simulink model "ARINC429_BNR"  (R2020b)
settings: Solver=VariableStepAuto  StartTime=0.0  StopTime=10.0  RelTol=1e-3
libraries: Bibavion x1
(part 1 of 3)
settings Model: Creator=Nicolas  LastModifiedBy=rolla

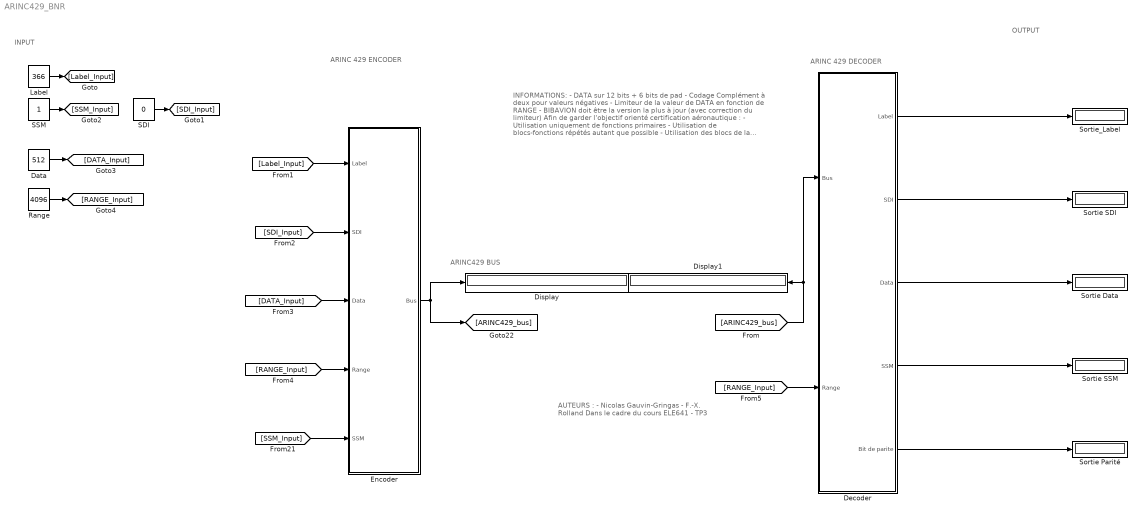
== system ARINC429_BNR ==
  note: AUTEURS :
      | - Nicolas Gauvin-Gringas
      | - F.-X. Rolland
      |
      | Dans le cadre du cours ELE641 - TP3
  note: INFORMATIONS:
      | - DATA sur 12 bits + 6 bits de pad
      | - Codage Complément à deux pour valeurs négatives
      | - Limiteur de la valeur de DATA en fonction de RANGE
      | - BIBAVION doit être la version la plus à jour (avec correction du limiteur)
      |
      | Afin de garder l'objectif orienté certification aéronautique :
      | - Utilisation uniquement de fonctions primaires
      | - Utilisation de blocs-fonctions répétés autant que possible
      | - Utilisation des blocs de la fonction BIBAVION partout la où possible
  note: ARINC 429 DECODER
  note: ARINC 429 ENCODER
  note: ARINC429 BUS
  note: OUTPUT
  note: INPUT
  Data : Constant  Value=512  OutDataTypeStr=int32  SampleTime=-1
  Decoder : Subsystem
  Display : Display
      settings: Format=binary (Stored Integer)
  Display1 : Display
      settings: Format=binary (Stored Integer)
  Encoder : Subsystem
  Label : Constant  Value=366  OutDataTypeStr=uint32  SampleTime=-1
  Range : Constant  Value=4096  OutDataTypeStr=uint32  SampleTime=-1
  SDI : Constant  Value=0  OutDataTypeStr=uint32  SampleTime=-1
  SSM : Constant  OutDataTypeStr=uint32  SampleTime=-1
  Sortie Data : Display
  Sortie Parité : Display
  Sortie SDI : Display
  Sortie SSM : Display
  Sortie_Label : Display
  wires:
  [ARINC429_bus] -> Decoder/1(Bus), Display1/1
  Label/1 -> [Label_Input]
  SDI/1 -> [SDI_Input]
  SSM/1 -> [SSM_Input]
  Decoder/1(Label) -> Sortie_Label/1
  [Label_Input] -> Encoder/1(Label)
  Encoder/1(Bus) -> Display/1, [ARINC429_bus]
  [SDI_Input] -> Encoder/2(SDI)
  [SSM_Input] -> Encoder/5(SSM)
  Decoder/2(SDI) -> Sortie SDI/1
  Decoder/3(Data) -> Sortie Data/1
  Decoder/4(SSM) -> Sortie SSM/1
  Decoder/5(Bit de parite) -> Sortie Parité/1
  Range/1 -> [RANGE_Input]
  [RANGE_Input] -> Encoder/4(Range)
  Data/1 -> [DATA_Input]
  [DATA_Input] -> Encoder/3(Data)
  [RANGE_Input] -> Decoder/2(Range)

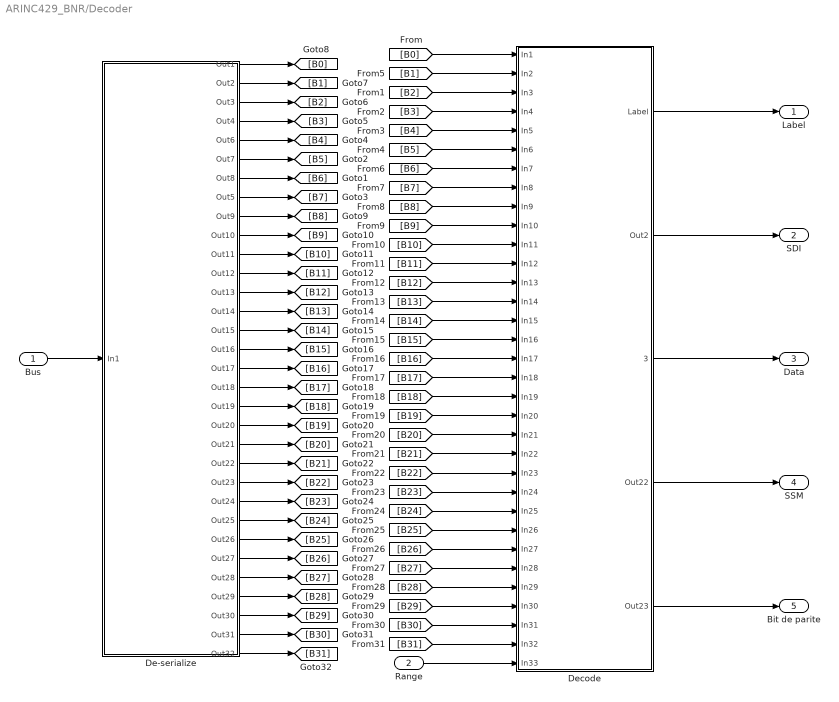
== system ARINC429_BNR/Decoder ==
  Bus : Inport
  Range : Inport  Port=2
  De-serialize : Subsystem
  Decode : Subsystem
  Label : Outport
  SDI : Outport  Port=2
  Data : Outport  Port=3
  SSM : Outport  Port=4
  Bit de parite : Outport  Port=5
  wires:
  De-serialize/6(Out7) -> [B5]
  De-serialize/1(Out1) -> [B0]
  De-serialize/7(Out8) -> [B6]
  De-serialize/5(Out6) -> [B4]
  De-serialize/3(Out3) -> [B2]
  De-serialize/2(Out2) -> [B1]
  De-serialize/4(Out4) -> [B3]
  De-serialize/8(Out5) -> [B7]
  Bus/1 -> De-serialize/1(In1)
  [B1] -> Decode/2(In2)
  [B0] -> Decode/1(In1)
  [B2] -> Decode/3(In3)
  [B3] -> Decode/4(In4)
  [B4] -> Decode/5(In5)
  [B5] -> Decode/6(In6)
  [B6] -> Decode/7(In7)
  [B7] -> Decode/8(In8)
  De-serialize/9(Out9) -> [B8]
  De-serialize/10(Out10) -> [B9]
  De-serialize/11(Out11) -> [B10]
  De-serialize/12(Out12) -> [B11]
  De-serialize/13(Out13) -> [B12]
  De-serialize/14(Out14) -> [B13]
  De-serialize/15(Out15) -> [B14]
  De-serialize/16(Out16) -> [B15]
  De-serialize/17(Out17) -> [B16]
  De-serialize/18(Out18) -> [B17]
  De-serialize/19(Out19) -> [B18]
  De-serialize/20(Out20) -> [B19]
  De-serialize/21(Out21) -> [B20]
  De-serialize/22(Out22) -> [B21]
  De-serialize/23(Out23) -> [B22]
  De-serialize/24(Out24) -> [B23]
  De-serialize/25(Out25) -> [B24]
  De-serialize/26(Out26) -> [B25]
  De-serialize/27(Out27) -> [B26]
  De-serialize/28(Out28) -> [B27]
  De-serialize/29(Out29) -> [B28]
  De-serialize/30(Out30) -> [B29]
  De-serialize/31(Out31) -> [B30]
  De-serialize/32(Out32) -> [B31]
  [B8] -> Decode/9(In9)
  [B9] -> Decode/10(In10)
  [B10] -> Decode/11(In11)
  [B11] -> Decode/12(In12)
  [B12] -> Decode/13(In13)
  [B13] -> Decode/14(In14)
  [B14] -> Decode/15(In15)
  [B15] -> Decode/16(In16)
  [B16] -> Decode/17(In17)
  [B17] -> Decode/18(In18)
  [B18] -> Decode/19(In19)
  [B19] -> Decode/20(In20)
  [B20] -> Decode/21(In21)
  [B21] -> Decode/22(In22)
  [B22] -> Decode/23(In23)
  [B23] -> Decode/24(In24)
  [B24] -> Decode/25(In25)
  [B25] -> Decode/26(In26)
  [B26] -> Decode/27(In27)
  [B27] -> Decode/28(In28)
  [B28] -> Decode/29(In29)
  [B29] -> Decode/30(In30)
  [B30] -> Decode/31(In31)
  [B31] -> Decode/32(In32)
  Decode/4(Out22) -> SSM/1
  Decode/5(Out23) -> Bit de parite/1
  Decode/2(Out2) -> SDI/1
  Decode/3(3) -> Data/1
  Range/1 -> Decode/33(In33)
  Decode/1(Label) -> Label/1

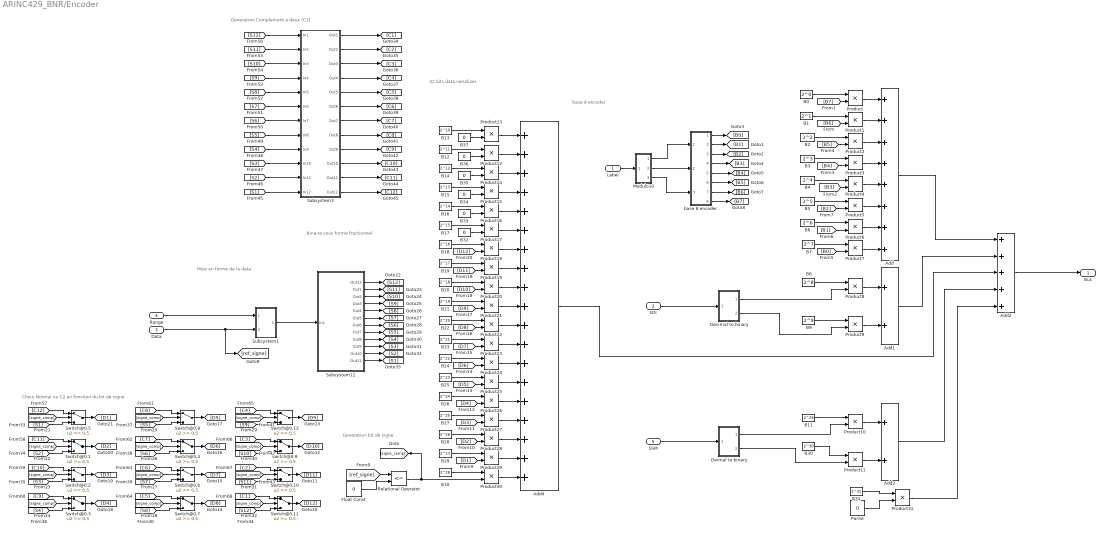
== system ARINC429_BNR/Encoder ==
  note: Generation Complement à deux (C2)
  note: Choix Normal ou C2 en fonction du bit de signe
  note: Generation bit de signe
  note: Binaire sous forme fractionnel
  note: Mise en forme de la data
  note: base 8 encoder
  note: 32 bits data serializer
  Label : Inport
  SDI : Inport  Port=2
  Data : Inport  Port=3
  Range : Inport  Port=4
  SSM : Inport  Port=5
  Add : Sum  Inputs=++++++++  AccumDataTypeStr=uint32  OutDataTypeStr=uint32
  Add1 : Sum  AccumDataTypeStr=uint32  OutDataTypeStr=uint32
  Add2 : Sum  Inputs=+++++  AccumDataTypeStr=uint32  OutDataTypeStr=uint32
  Add3 : Sum  AccumDataTypeStr=uint32  OutDataTypeStr=uint32
  Add4 : Sum  Inputs=+++++++++++++++++++  AccumDataTypeStr=uint32  OutDataTypeStr=uint32
  B0 : Constant  Value=2^0  OutDataTypeStr=single
  B1 : Constant  Value=2^1  OutDataTypeStr=single
  B10 : Constant  Value=2^28  OutDataTypeStr=single
  B11 : Constant  Value=2^29  OutDataTypeStr=single
  B12 : Constant  Value=2^11  OutDataTypeStr=single
  B13 : Constant  Value=2^10  OutDataTypeStr=single
  B14 : Constant  Value=2^12  OutDataTypeStr=single
  B15 : Constant  Value=2^13  OutDataTypeStr=single
  B16 : Constant  Value=2^14  OutDataTypeStr=single
  B17 : Constant  Value=2^15  OutDataTypeStr=single
  B18 : Constant  Value=2^16  OutDataTypeStr=single
  B19 : Constant  Value=2^17  OutDataTypeStr=single
  B2 : Constant  Value=2^2  OutDataTypeStr=single
  B20 : Constant  Value=2^18  OutDataTypeStr=single
  B21 : Constant  Value=2^19  OutDataTypeStr=single
  B22 : Constant  Value=2^20  OutDataTypeStr=single
  B23 : Constant  Value=2^21  OutDataTypeStr=single
  B24 : Constant  Value=2^22  OutDataTypeStr=single
  B25 : Constant  Value=2^23  OutDataTypeStr=single
  B26 : Constant  Value=2^24  OutDataTypeStr=single
  B27 : Constant  Value=2^25  OutDataTypeStr=single
  B28 : Constant  Value=2^26  OutDataTypeStr=single
  B29 : Constant  Value=2^27  OutDataTypeStr=single
  B3 : Constant  Value=2^3  OutDataTypeStr=single
  B30 : Constant  Value=2^30  OutDataTypeStr=single
  B31 : Constant  Value=2^31  OutDataTypeStr=single
  B{32..37} (6 alike) : Constant  Value=0  OutDataTypeStr=single
  B4 : Constant  Value=2^4  OutDataTypeStr=single
  B5 : Constant  Value=2^5  OutDataTypeStr=single
  B6 : Constant  Value=2^6  OutDataTypeStr=single
  B7 : Constant  Value=2^7  OutDataTypeStr=single
  B8 : Constant  Value=2^8  OutDataTypeStr=single
  B9 : Constant  Value=2^9  OutDataTypeStr=single
  Decimal to binary : Subsystem
  Deimal to binary : Subsystem
  Float Const : Constant  Value=0  OutDataTypeStr=uint32
  "Modulo10 " : Subsystem
  Parité : Constant  Value=0  OutDataTypeStr=boolean
  Product{,1..29,31} (31 alike) : Product
  Product30 : Product  OutDataTypeStr=single
  Relational Operator : RelationalOperator  Operator=<=  OutDataTypeStr=boolean  RndMeth=Nearest
  Subsystem1 : Subsystem
  Subsystem12 : Subsystem
  Subsystem3 : Subsystem
  Switch@0.{1..12} (12 alike) : Switch  Threshold=0.5
  base 8 encoder : Subsystem
  Bus : Outport
  wires:
  base 8 encoder/4(Out4) -> [B3]
  B5/1 -> Product5/1
  [B0] -> Product7/2
  B2/1 -> Product2/1
  [B5] -> Product2/2
  [B3] -> Product4/2
  "Modulo10 "/2(Out2) -> base 8 encoder/2(In2)
  "Modulo10 "/3(Out3) -> base 8 encoder/3(In3)
  B0/1 -> Product/1
  Product3/1 -> Add/4
  [B7] -> Product/2
  Product4/1 -> Add/5
  base 8 encoder/5(Out5) -> [B4]
  base 8 encoder/8(Out8) -> [B7]
  [B6] -> Product1/2
  B1/1 -> Product1/1
  [B4] -> Product3/2
  B4/1 -> Product4/1
  base 8 encoder/3(Out3) -> [B2]
  Product/1 -> Add/1
  Product5/1 -> Add/6
  Product6/1 -> Add/7
  base 8 encoder/1(Out1) -> [B0]
  [B1] -> Product6/2
  base 8 encoder/7(Out7) -> [B6]
  Product2/1 -> Add/3
  B3/1 -> Product3/1
  Label/1 -> "Modulo10 "/1(In1)
  Product7/1 -> Add/8
  Product1/1 -> Add/2
  B6/1 -> Product6/1
  B7/1 -> Product7/1
  "Modulo10 "/1(Out1) -> base 8 encoder/1(In1)
  base 8 encoder/6(Out6) -> [B5]
  [B2] -> Product5/2
  base 8 encoder/2(Out2) -> [B1]
  Product9/1 -> Add1/2
  Product8/1 -> Add1/1
  B9/1 -> Product9/1
  B8/1 -> Product8/1
  Product10/1 -> Add3/1
  Product11/1 -> Add3/2
  B13/1 -> Product13/1
  B12/1 -> Product12/1
  B14/1 -> Product14/1
  B15/1 -> Product15/1
  B16/1 -> Product16/1
  B17/1 -> Product17/1
  B18/1 -> Product18/1
  B19/1 -> Product19/1
  B20/1 -> Product20/1
  B21/1 -> Product21/1
  B22/1 -> Product22/1
  B23/1 -> Product23/1
  B24/1 -> Product24/1
  B25/1 -> Product25/1
  B26/1 -> Product26/1
  B27/1 -> Product27/1
  B28/1 -> Product28/1
  B29/1 -> Product29/1
  SDI/1 -> Decimal to binary/1(In1)
  Decimal to binary/1(Out1) -> Product8/2
  Decimal to binary/2(Out2) -> Product9/2
  SSM/1 -> Deimal to binary/1(In1)
  Deimal to binary/1(Out1) -> Product10/2
  Deimal to binary/2(Out2) -> Product11/2
  B31/1 -> Product31/1
  Parité/1 -> Product31/2
  B11/1 -> Product10/1
  Add2/1 -> Bus/1
  Add/1 -> Add2/1
  Add1/1 -> Add2/2
  Add4/1 -> Add2/3
  B30/1 -> Product11/1
  Add3/1 -> Add2/4
  Product31/1 -> Add2/5
  Float Const/1 -> Relational Operator/2
  B10/1 -> Product30/1
  Product30/1 -> Add4/19
  Relational Operator/1 -> Product30/2, [signe_comp]
  Product13/1 -> Add4/1
  Product12/1 -> Add4/2
  Product14/1 -> Add4/3
  Product15/1 -> Add4/4
  Product16/1 -> Add4/5
  Product17/1 -> Add4/6
  Product18/1 -> Add4/7
  Product19/1 -> Add4/8
  Product20/1 -> Add4/9
  Product21/1 -> Add4/10
  Product22/1 -> Add4/11
  Product23/1 -> Add4/12
  Product24/1 -> Add4/13
  Product25/1 -> Add4/14
  Product26/1 -> Add4/15
  Product27/1 -> Add4/16
  Product28/1 -> Add4/17
  Product29/1 -> Add4/18
  [ref_signe] -> Relational Operator/1
  [D1] -> Product29/2
  [D2] -> Product28/2
  [D3] -> Product27/2
  [D4] -> Product26/2
  [D5] -> Product25/2
  [D6] -> Product24/2
  [D7] -> Product23/2
  [D8] -> Product22/2
  [D9] -> Product21/2
  [D10] -> Product20/2
  [D11] -> Product19/2
  [D12] -> Product18/2
  B32/1 -> Product17/2
  B33/1 -> Product16/2
  B34/1 -> Product15/2
  B35/1 -> Product14/2
  B36/1 -> Product12/2
  B37/1 -> Product13/2
  Switch@0.11/1 -> [D12]
  Switch@0.10/1 -> [D11]
  Switch@0.7/1 -> [D8]
  Switch@0.6/1 -> [D7]
  Switch@0.3/1 -> [D4]
  Switch@0.2/1 -> [D3]
  Switch@0.5/1 -> [D1]
  Switch@0.1/1 -> [D2]
  Switch@0.4/1 -> [D6]
  Switch@0.8/1 -> [D5]
  Switch@0.12/1 -> [D9]
  Switch@0.9/1 -> [D10]
  [signe_comp] -> Switch@0.5/2
  [signe_comp] -> Switch@0.1/2
  [signe_comp] -> Switch@0.2/2
  [signe_comp] -> Switch@0.3/2
  [signe_comp] -> Switch@0.8/2
  [signe_comp] -> Switch@0.4/2
  [signe_comp] -> Switch@0.6/2
  [signe_comp] -> Switch@0.7/2
  [signe_comp] -> Switch@0.12/2
  [signe_comp] -> Switch@0.9/2
  [signe_comp] -> Switch@0.10/2
  [signe_comp] -> Switch@0.11/2
  Subsystem12/12(Out11) -> [S1]
  Subsystem12/11(Out10) -> [S2]
  Subsystem12/9(Out8) -> [S4]
  Subsystem12/8(Out7) -> [S5]
  Subsystem12/7(Out6) -> [S6]
  Subsystem12/6(Out5) -> [S7]
  Subsystem12/4(Out3) -> [S9]
  Subsystem12/3(Out2) -> [S10]
  Subsystem12/2(Out1) -> [S11]
  [S1] -> Switch@0.5/3
  [S2] -> Switch@0.1/3
  [S3] -> Switch@0.2/3
  [S4] -> Switch@0.3/3
  [S5] -> Switch@0.8/3
  [S6] -> Switch@0.4/3
  [S7] -> Switch@0.6/3
  [S8] -> Switch@0.7/3
  [S9] -> Switch@0.12/3
  [S10] -> Switch@0.9/3
  [S11] -> Switch@0.10/3
  [S12] -> Switch@0.11/3
  Subsystem12/1(Out12) -> [S12]
  Subsystem12/5(Out4) -> [S8]
  Subsystem12/10(Out9) -> [S3]
  [C12] -> Switch@0.5/1
  [C11] -> Switch@0.1/1
  [C10] -> Switch@0.2/1
  [C9] -> Switch@0.3/1
  [C8] -> Switch@0.8/1
  [C7] -> Switch@0.4/1
  [C6] -> Switch@0.6/1
  [C5] -> Switch@0.7/1
  [C4] -> Switch@0.12/1
  [C3] -> Switch@0.9/1
  [C2] -> Switch@0.10/1
  [C1] -> Switch@0.11/1
  Range/1 -> Subsystem1/1(In1)
  Data/1 -> [ref_signe], Subsystem1/2(In2)
  Subsystem1/1(Out1) -> Subsystem12/1(In1)
  [S12] -> Subsystem3/1(In1)
  [S11] -> Subsystem3/2(In2)
  [S10] -> Subsystem3/3(In3)
  [S9] -> Subsystem3/4(In4)
  [S8] -> Subsystem3/5(In5)
  [S7] -> Subsystem3/6(In6)
  [S6] -> Subsystem3/7(In7)
  [S5] -> Subsystem3/8(In8)
  [S4] -> Subsystem3/9(In9)
  [S3] -> Subsystem3/10(In10)
  [S2] -> Subsystem3/11(In11)
  [S1] -> Subsystem3/12(In12)
  Subsystem3/1(Out1) -> [C1]
  Subsystem3/2(Out2) -> [C2]
  Subsystem3/3(Out3) -> [C3]
  Subsystem3/4(Out4) -> [C4]
  Subsystem3/5(Out5) -> [C5]
  Subsystem3/6(Out6) -> [C6]
  Subsystem3/7(Out7) -> [C7]
  Subsystem3/8(Out8) -> [C8]
  Subsystem3/9(Out9) -> [C9]
  Subsystem3/10(Out10) -> [C10]
  Subsystem3/11(Out11) -> [C11]
  Subsystem3/12(Out12) -> [C12]

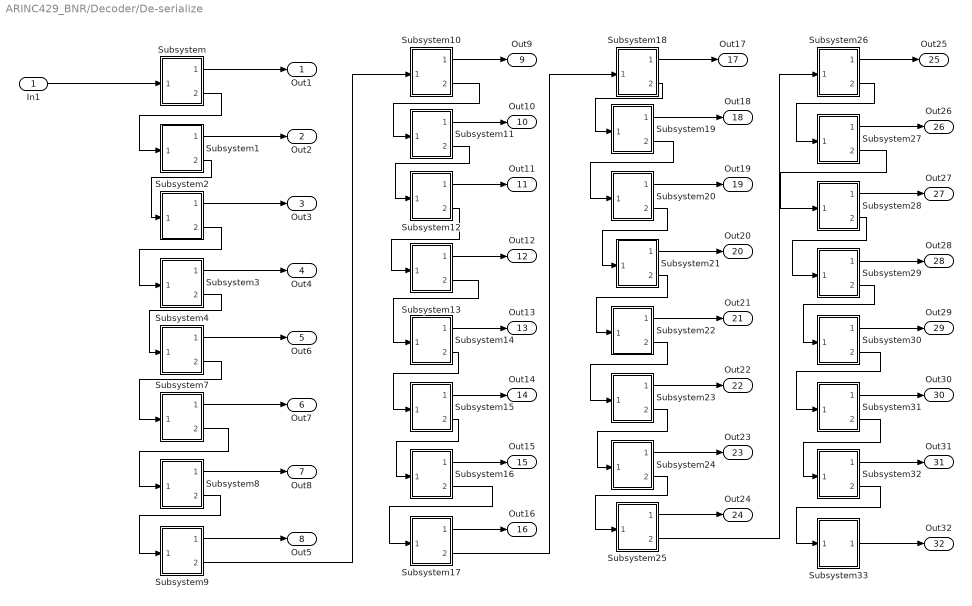
== system ARINC429_BNR/Decoder/De-serialize ==
  In1 : Inport
  Subsystem : Subsystem
  Subsystem1 : Subsystem
  Subsystem10 : Subsystem
  Subsystem11 : Subsystem
  Subsystem12 : Subsystem
  Subsystem13 : Subsystem
  Subsystem14 : Subsystem
  Subsystem15 : Subsystem
  Subsystem16 : Subsystem
  Subsystem17 : Subsystem
  Subsystem18 : Subsystem
  Subsystem19 : Subsystem
  Subsystem2 : Subsystem
  Subsystem20 : Subsystem
  Subsystem21 : Subsystem
  Subsystem22 : Subsystem
  Subsystem23 : Subsystem
  Subsystem24 : Subsystem
  Subsystem25 : Subsystem
  Subsystem26 : Subsystem
  Subsystem27 : Subsystem
  Subsystem28 : Subsystem
  Subsystem29 : Subsystem
  Subsystem3 : Subsystem
  Subsystem30 : Subsystem
  Subsystem31 : Subsystem
  Subsystem32 : Subsystem
  Subsystem33 : Subsystem
  Subsystem4 : Subsystem
  Subsystem7 : Subsystem
  Subsystem8 : Subsystem
  Subsystem9 : Subsystem
  Out1 : Outport
  Out2 : Outport  Port=2
  Out3 : Outport  Port=3
  Out4 : Outport  Port=4
  Out6 : Outport  Port=5
  Out7 : Outport  Port=6
  Out8 : Outport  Port=7
  Out5 : Outport  Port=8
  Out9 : Outport  Port=9
  Out10 : Outport  Port=10
  Out11 : Outport  Port=11
  Out12 : Outport  Port=12
  Out13 : Outport  Port=13
  Out14 : Outport  Port=14
  Out15 : Outport  Port=15
  Out16 : Outport  Port=16
  Out17 : Outport  Port=17
  Out18 : Outport  Port=18
  Out19 : Outport  Port=19
  Out20 : Outport  Port=20
  Out21 : Outport  Port=21
  Out22 : Outport  Port=22
  Out23 : Outport  Port=23
  Out24 : Outport  Port=24
  Out25 : Outport  Port=25
  Out26 : Outport  Port=26
  Out27 : Outport  Port=27
  Out28 : Outport  Port=28
  Out29 : Outport  Port=29
  Out30 : Outport  Port=30
  Out31 : Outport  Port=31
  Out32 : Outport  Port=32
  wires:
  Subsystem/1(Out1) -> Out1/1
  Subsystem1/1(Out1) -> Out2/1
  Subsystem1/2(Out2) -> Subsystem2/1(In1)
  Subsystem2/2(Out2) -> Subsystem3/1(In1)
  Subsystem3/2(Out2) -> Subsystem4/1(In1)
  Subsystem2/1(Out1) -> Out3/1
  Subsystem3/1(Out1) -> Out4/1
  Subsystem4/2(Out2) -> Subsystem7/1(In1)
  Subsystem4/1(Out1) -> Out6/1
  Subsystem7/1(Out1) -> Out7/1
  Subsystem8/1(Out1) -> Out8/1
  Subsystem10/2(Out2) -> Subsystem11/1(In1)
  Subsystem12/2(Out2) -> Subsystem13/1(In1)
  Subsystem14/2(Out2) -> Subsystem15/1(In1)
  Subsystem11/2(Out2) -> Subsystem12/1(In1)
  Subsystem15/2(Out2) -> Subsystem16/1(In1)
  Subsystem16/2(Out2) -> Subsystem17/1(In1)
  Subsystem23/2(Out2) -> Subsystem24/1(In1)
  Subsystem18/2(Out2) -> Subsystem19/1(In1)
  Subsystem21/2(Out2) -> Subsystem22/1(In1)
  Subsystem22/2(Out2) -> Subsystem23/1(In1)
  Subsystem19/2(Out2) -> Subsystem20/1(In1)
  Subsystem20/2(Out2) -> Subsystem21/1(In1)
  Subsystem24/2(Out2) -> Subsystem25/1(In1)
  Subsystem29/2(Out2) -> Subsystem30/1(In1)
  Subsystem27/2(Out2) -> Subsystem28/1(In1)
  Subsystem28/2(Out2) -> Subsystem29/1(In1)
  Subsystem26/2(Out2) -> Subsystem27/1(In1)
  Subsystem9/1(Out1) -> Out5/1
  Subsystem17/2(Out2) -> Subsystem18/1(In1)
  Subsystem25/2(Out2) -> Subsystem26/1(In1)
  Subsystem9/2(Out2) -> Subsystem10/1(In1)
  Subsystem10/1(Out1) -> Out9/1
  Subsystem11/1(Out1) -> Out10/1
  Subsystem12/1(Out1) -> Out11/1
  Subsystem13/1(Out1) -> Out12/1
  Subsystem14/1(Out1) -> Out13/1
  Subsystem15/1(Out1) -> Out14/1
  Subsystem16/1(Out1) -> Out15/1
  Subsystem17/1(Out1) -> Out16/1
  Subsystem18/1(Out1) -> Out17/1
  Subsystem19/1(Out1) -> Out18/1
  Subsystem20/1(Out1) -> Out19/1
  Subsystem21/1(Out1) -> Out20/1
  Subsystem22/1(Out1) -> Out21/1
  Subsystem23/1(Out1) -> Out22/1
  Subsystem24/1(Out1) -> Out23/1
  Subsystem25/1(Out1) -> Out24/1
  Subsystem26/1(Out1) -> Out25/1
  Subsystem27/1(Out1) -> Out26/1
  Subsystem28/1(Out1) -> Out27/1
  Subsystem29/1(Out1) -> Out28/1
  Subsystem33/1(Out1) -> Out32/1
  Subsystem30/2(Out2) -> Subsystem31/1(In1)
  Subsystem31/2(Out2) -> Subsystem32/1(In1)
  Subsystem32/2(Out2) -> Subsystem33/1(In1)
  Subsystem32/1(Out1) -> Out31/1
  Subsystem31/1(Out1) -> Out30/1
  Subsystem30/1(Out1) -> Out29/1
  Subsystem7/2(Out2) -> Subsystem8/1(In1)
  Subsystem8/2(Out2) -> Subsystem9/1(In1)
  Subsystem/2(Out2) -> Subsystem1/1(In1)
  In1/1 -> Subsystem/1(In1)
  Subsystem13/2(Out2) -> Subsystem14/1(In1)

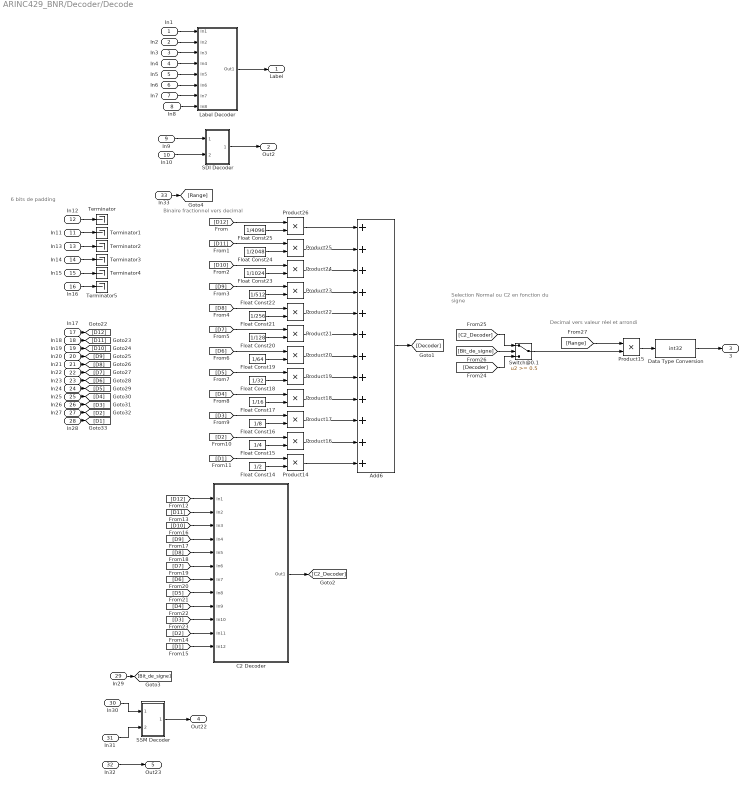
== system ARINC429_BNR/Decoder/Decode ==
  note: 6 bits de padding
  note: Selection Normal ou C2
      | en fonction du signe
  note: Decimal vers valeur réel et arrondi
  note: Binaire fractionnel vers decimal
  In1 : Inport
  In2 : Inport  Port=2
  In3 : Inport  Port=3
  In4 : Inport  Port=4
  In5 : Inport  Port=5
  In6 : Inport  Port=6
  In7 : Inport  Port=7
  In8 : Inport  Port=8
  In9 : Inport  Port=9
  In10 : Inport  Port=10
  In11 : Inport  Port=11
  In12 : Inport  Port=12
  In13 : Inport  Port=13
  In14 : Inport  Port=14
  In15 : Inport  Port=15
  In16 : Inport  Port=16
  In17 : Inport  Port=17
  In18 : Inport  Port=18
  In19 : Inport  Port=19
  In20 : Inport  Port=20
  In21 : Inport  Port=21
  In22 : Inport  Port=22
  In23 : Inport  Port=23
  In24 : Inport  Port=24
  In25 : Inport  Port=25
  In26 : Inport  Port=26
  In27 : Inport  Port=27
  In28 : Inport  Port=28
  In29 : Inport  Port=29
  In30 : Inport  Port=30
  In31 : Inport  Port=31
  In32 : Inport  Port=32
  In33 : Inport  Port=33
  Add6 : Sum  Inputs=++++++++++++
  C2 Decoder : Subsystem
  Data Type Conversion : DataTypeConversion  OutDataTypeStr=int32  RndMeth=Nearest
  Float Const14 : Constant  Value=1/2  OutDataTypeStr=single
  Float Const15 : Constant  Value=1/4  OutDataTypeStr=single
  Float Const16 : Constant  Value=1/8  OutDataTypeStr=single
  Float Const17 : Constant  Value=1/16  OutDataTypeStr=single
  Float Const18 : Constant  Value=1/32  OutDataTypeStr=single
  Float Const19 : Constant  Value=1/64  OutDataTypeStr=single
  Float Const20 : Constant  Value=1/128  OutDataTypeStr=single
  Float Const21 : Constant  Value=1/256  OutDataTypeStr=single
  Float Const22 : Constant  Value=1/512  OutDataTypeStr=single
  Float Const23 : Constant  Value=1/1024  OutDataTypeStr=single
  Float Const24 : Constant  Value=1/2048  OutDataTypeStr=single
  Float Const25 : Constant  Value=1/4096  OutDataTypeStr=single
  Label Decoder : Subsystem
  Product{14..26} (13 alike) : Product
  SDI Decoder : Subsystem
  SSM Decoder : Subsystem
  Switch@0.1 : Switch  Threshold=0.5
  Terminator{,1..5} (6 alike) : Terminator
  Label : Outport
  Out2 : Outport  Port=2
  3 : Outport  Port=3
  Out22 : Outport  Port=4
  Out23 : Outport  Port=5
  wires:
  In32/1 -> Out23/1
  Float Const14/1 -> Product14/2
  Float Const15/1 -> Product16/2
  Float Const16/1 -> Product17/2
  Float Const17/1 -> Product18/2
  Float Const18/1 -> Product19/2
  Float Const19/1 -> Product20/2
  Float Const20/1 -> Product21/2
  Float Const21/1 -> Product22/2
  Float Const22/1 -> Product23/2
  Float Const23/1 -> Product24/2
  Float Const24/1 -> Product25/2
  Float Const25/1 -> Product26/2
  Product14/1 -> Add6/12
  Product16/1 -> Add6/11
  Product17/1 -> Add6/10
  Product18/1 -> Add6/9
  Product19/1 -> Add6/8
  Product20/1 -> Add6/7
  Product21/1 -> Add6/6
  Product22/1 -> Add6/5
  Product23/1 -> Add6/4
  Product24/1 -> Add6/3
  Product25/1 -> Add6/2
  Product26/1 -> Add6/1
  In12/1 -> Terminator/1
  In11/1 -> Terminator1/1
  In13/1 -> Terminator2/1
  In15/1 -> Terminator4/1
  In16/1 -> Terminator5/1
  In14/1 -> Terminator3/1
  Product15/1 -> Data Type Conversion/1
  Data Type Conversion/1 -> 3/1
  In28/1 -> [D1]
  In27/1 -> [D2]
  In17/1 -> [D12]
  In18/1 -> [D11]
  In19/1 -> [D10]
  In20/1 -> [D9]
  In21/1 -> [D8]
  In22/1 -> [D7]
  In23/1 -> [D6]
  In24/1 -> [D5]
  In25/1 -> [D4]
  In26/1 -> [D3]
  [D12] -> Product26/1
  [D11] -> Product25/1
  [D10] -> Product24/1
  [D9] -> Product23/1
  [D8] -> Product22/1
  [D7] -> Product21/1
  [D6] -> Product20/1
  [D5] -> Product19/1
  [D4] -> Product18/1
  [D3] -> Product17/1
  [D2] -> Product16/1
  [D1] -> Product14/1
  [D12] -> C2 Decoder/1(In1)
  [D11] -> C2 Decoder/2(In2)
  [D10] -> C2 Decoder/3(In3)
  [D9] -> C2 Decoder/4(In4)
  [D8] -> C2 Decoder/5(In5)
  [D7] -> C2 Decoder/6(In6)
  [D6] -> C2 Decoder/7(In7)
  [D5] -> C2 Decoder/8(In8)
  [D4] -> C2 Decoder/9(In9)
  [D3] -> C2 Decoder/10(In10)
  [D2] -> C2 Decoder/11(In11)
  [D1] -> C2 Decoder/12(In12)
  Switch@0.1/1 -> Product15/2
  Add6/1 -> [Decoder]
  C2 Decoder/1(Out1) -> [C2_Decoder]
  [C2_Decoder] -> Switch@0.1/1
  [Decoder] -> Switch@0.1/3
  In29/1 -> [Bit_de_signe]
  [Bit_de_signe] -> Switch@0.1/2
  In33/1 -> [Range]
  [Range] -> Product15/1
  In1/1 -> Label Decoder/1(In1)
  In2/1 -> Label Decoder/2(In2)
  In3/1 -> Label Decoder/3(In3)
  In4/1 -> Label Decoder/4(In4)
  In5/1 -> Label Decoder/5(In5)
  In6/1 -> Label Decoder/6(In6)
  In7/1 -> Label Decoder/7(In7)
  In8/1 -> Label Decoder/8(In8)
  Label Decoder/1(Out1) -> Label/1
  In9/1 -> SDI Decoder/1(In1)
  In10/1 -> SDI Decoder/2(In2)
  SDI Decoder/1(Out1) -> Out2/1
  In30/1 -> SSM Decoder/1(In1)
  In31/1 -> SSM Decoder/2(In2)
  SSM Decoder/1(Out1) -> Out22/1

== system ARINC429_BNR/Encoder/Decimal to binary ==
  In1 : Inport
  OR : Logic  Operator=OR  IconShape=distinctive  AllPortsSameDT=off  OutDataTypeStr=boolean
  OR1 : Logic  Operator=OR  IconShape=distinctive  AllPortsSameDT=off  OutDataTypeStr=boolean
  Relational Operator{,1..3} (4 alike) : RelationalOperator  Operator===  OutDataTypeStr=boolean  RndMeth=Nearest
  uint32 constant : Constant  OutDataTypeStr=uint32  SampleTime=-1
  uint32 constant1 : Constant  Value=3  OutDataTypeStr=uint32  SampleTime=-1
  uint32 constant2 : Constant  Value=2  OutDataTypeStr=uint32  SampleTime=-1
  uint32 constant3 : Constant  Value=3  OutDataTypeStr=uint32  SampleTime=-1
  Out1 : Outport
  Out2 : Outport  Port=2
  wires:
  uint32 constant1/1 -> Relational Operator1/2
  Relational Operator1/1 -> OR/2
  uint32 constant3/1 -> Relational Operator3/2
  Relational Operator/1 -> OR/1
  uint32 constant2/1 -> Relational Operator2/2
  In1/1 -> Relational Operator/1, Relational Operator1/1, Relational Operator3/1, Relational Operator2/1
  Relational Operator3/1 -> OR1/2
  uint32 constant/1 -> Relational Operator/2
  Relational Operator2/1 -> OR1/1
  OR1/1 -> Out2/1
  OR/1 -> Out1/1

== system ARINC429_BNR/Encoder/Deimal to binary ==
  In1 : Inport
  OR : Logic  Operator=OR  IconShape=distinctive  AllPortsSameDT=off  OutDataTypeStr=boolean
  OR1 : Logic  Operator=OR  IconShape=distinctive  AllPortsSameDT=off  OutDataTypeStr=boolean
  Relational Operator{,1..3} (4 alike) : RelationalOperator  Operator===  OutDataTypeStr=boolean  RndMeth=Nearest
  uint32 constant : Constant  OutDataTypeStr=uint32  SampleTime=-1
  uint32 constant1 : Constant  Value=3  OutDataTypeStr=uint32  SampleTime=-1
  uint32 constant2 : Constant  Value=2  OutDataTypeStr=uint32  SampleTime=-1
  uint32 constant3 : Constant  Value=3  OutDataTypeStr=uint32  SampleTime=-1
  Out1 : Outport
  Out2 : Outport  Port=2
  wires:
  uint32 constant1/1 -> Relational Operator1/2
  Relational Operator1/1 -> OR/2
  uint32 constant3/1 -> Relational Operator3/2
  Relational Operator/1 -> OR/1
  uint32 constant2/1 -> Relational Operator2/2
  In1/1 -> Relational Operator/1, Relational Operator1/1, Relational Operator3/1, Relational Operator2/1
  Relational Operator3/1 -> OR1/2
  uint32 constant/1 -> Relational Operator/2
  Relational Operator2/1 -> OR1/1
  OR1/1 -> Out2/1
  OR/1 -> Out1/1

== system ARINC429_BNR/Encoder/Modulo10  ==
  In1 : Inport
  Subsystem : Subsystem
  Subsystem1 : Subsystem
  Subsystem2 : Subsystem
  Out1 : Outport
  Out2 : Outport  Port=2
  Out3 : Outport  Port=3
  wires:
  In1/1 -> Subsystem/1(In1)
  Subsystem/1(Out1) -> Out1/1
  Subsystem/2(Out2) -> Subsystem1/1(In1)
  Subsystem1/1(Out1) -> Out2/1
  Subsystem1/2(Out2) -> Subsystem2/1(In1)
  Subsystem2/1(Out1) -> Out3/1

== system ARINC429_BNR/Encoder/Subsystem1 ==
  In1 : Inport
  In2 : Inport  Port=2
  Abs1 : Abs
  Abs2 : Abs
  Data Type Conversion : DataTypeConversion  OutDataTypeStr=single
  Data Type Conversion1 : DataTypeConversion  OutDataTypeStr=single
  Divide : Product  Inputs=*/
  Gain : Gain  Gain=-1
  Saturation : Bibavion/Discontinuities/Saturation
      settings: SourceProductName=Bibavion P20
  Out1 : Outport
  wires:
  Divide/1 -> Abs2/1
  Gain/1 -> Saturation/3
  Abs1/1 -> Saturation/2, Divide/2, Gain/1
  Data Type Conversion1/1 -> Saturation/1
  Data Type Conversion/1 -> Abs1/1
  Saturation/1 -> Divide/1
  In1/1 -> Data Type Conversion/1
  Abs2/1 -> Out1/1
  In2/1 -> Data Type Conversion1/1

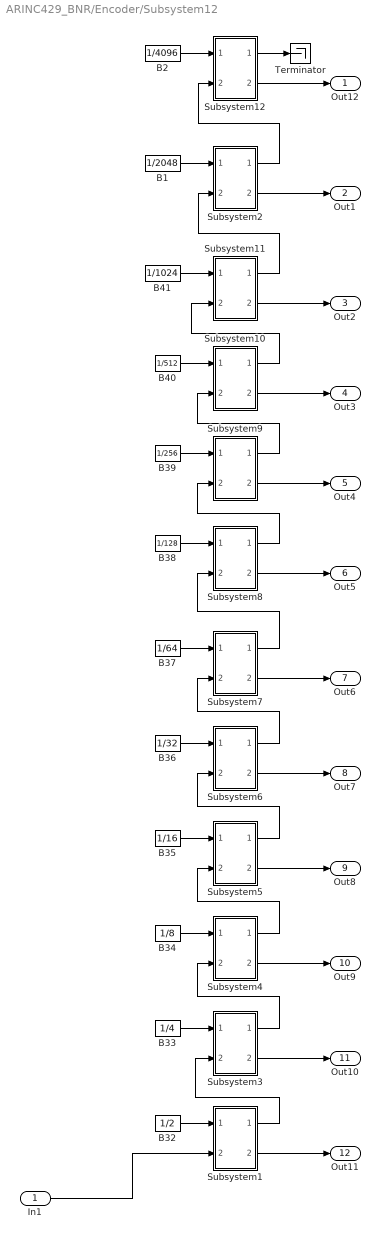
== system ARINC429_BNR/Encoder/Subsystem12 ==
  In1 : Inport
  B1 : Constant  Value=1/2048  OutDataTypeStr=single
  B2 : Constant  Value=1/4096  OutDataTypeStr=single
  B32 : Constant  Value=1/2  OutDataTypeStr=single
  B33 : Constant  Value=1/4  OutDataTypeStr=single
  B34 : Constant  Value=1/8  OutDataTypeStr=single
  B35 : Constant  Value=1/16  OutDataTypeStr=single
  B36 : Constant  Value=1/32  OutDataTypeStr=single
  B37 : Constant  Value=1/64  OutDataTypeStr=single
  B38 : Constant  Value=1/128  OutDataTypeStr=single
  B39 : Constant  Value=1/256  OutDataTypeStr=single
  B40 : Constant  Value=1/512  OutDataTypeStr=single
  B41 : Constant  Value=1/1024  OutDataTypeStr=single
  Subsystem1 : Subsystem
  Subsystem10 : Subsystem
  Subsystem11 : Subsystem
  Subsystem12 : Subsystem
  Subsystem2 : Subsystem
  Subsystem3 : Subsystem
  Subsystem4 : Subsystem
  Subsystem5 : Subsystem
  Subsystem6 : Subsystem
  Subsystem7 : Subsystem
  Subsystem8 : Subsystem
  Subsystem9 : Subsystem
  Terminator : Terminator
  Out12 : Outport
  Out1 : Outport  Port=2
  Out2 : Outport  Port=3
  Out3 : Outport  Port=4
  Out4 : Outport  Port=5
  Out5 : Outport  Port=6
  Out6 : Outport  Port=7
  Out7 : Outport  Port=8
  Out8 : Outport  Port=9
  Out9 : Outport  Port=10
  Out10 : Outport  Port=11
  Out11 : Outport  Port=12
  wires:
  Subsystem5/2(Out1) -> Out8/1
  B34/1 -> Subsystem4/1(In1)
  B38/1 -> Subsystem8/1(In1)
  B39/1 -> Subsystem9/1(In1)
  Subsystem3/1(Out2) -> Subsystem4/2(In2)
  B37/1 -> Subsystem7/1(In1)
  Subsystem6/1(Out2) -> Subsystem7/2(In2)
  B35/1 -> Subsystem5/1(In1)
  Subsystem9/1(Out2) -> Subsystem10/2(In2)
  Subsystem7/2(Out1) -> Out6/1
  Subsystem8/1(Out2) -> Subsystem9/2(In2)
  Subsystem5/1(Out2) -> Subsystem6/2(In2)
  In1/1 -> Subsystem1/2(In2)
  Subsystem4/1(Out2) -> Subsystem5/2(In2)
  Subsystem1/2(Out1) -> Out11/1
  B33/1 -> Subsystem3/1(In1)
  B41/1 -> Subsystem11/1(In1)
  Subsystem1/1(Out2) -> Subsystem3/2(In2)
  Subsystem6/2(Out1) -> Out7/1
  B40/1 -> Subsystem10/1(In1)
  B32/1 -> Subsystem1/1(In1)
  B36/1 -> Subsystem6/1(In1)
  Subsystem7/1(Out2) -> Subsystem8/2(In2)
  Subsystem10/1(Out2) -> Subsystem11/2(In2)
  Subsystem9/2(Out1) -> Out4/1
  Subsystem8/2(Out1) -> Out5/1
  Subsystem4/2(Out1) -> Out9/1
  Subsystem10/2(Out1) -> Out3/1
  Subsystem3/2(Out1) -> Out10/1
  B1/1 -> Subsystem2/1(In1)
  Subsystem2/2(Out1) -> Out1/1
  Subsystem11/1(Out2) -> Subsystem2/2(In2)
  Subsystem12/2(Out1) -> Out12/1
  Subsystem2/1(Out2) -> Subsystem12/2(In2)
  B2/1 -> Subsystem12/1(In1)
  Subsystem12/1(Out2) -> Terminator/1
  Subsystem11/2(Out1) -> Out2/1

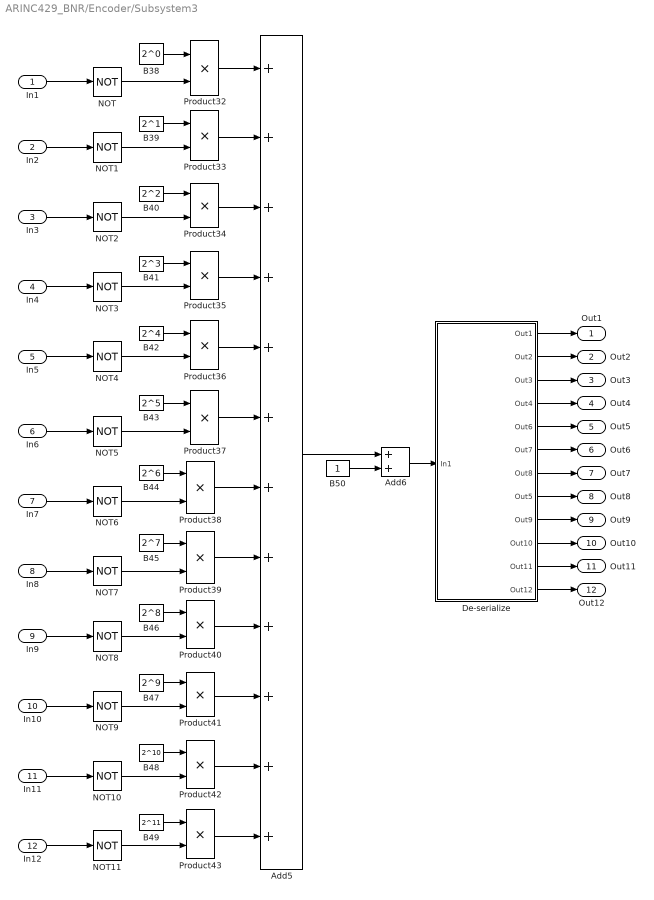
== system ARINC429_BNR/Encoder/Subsystem3 ==
  In1 : Inport
  In2 : Inport  Port=2
  In3 : Inport  Port=3
  In4 : Inport  Port=4
  In5 : Inport  Port=5
  In6 : Inport  Port=6
  In7 : Inport  Port=7
  In8 : Inport  Port=8
  In9 : Inport  Port=9
  In10 : Inport  Port=10
  In11 : Inport  Port=11
  In12 : Inport  Port=12
  Add5 : Sum  Inputs=++++++++++++  AccumDataTypeStr=uint32  OutDataTypeStr=uint32
  Add6 : Sum
  B38 : Constant  Value=2^0  OutDataTypeStr=single
  B39 : Constant  Value=2^1  OutDataTypeStr=single
  B40 : Constant  Value=2^2  OutDataTypeStr=single
  B41 : Constant  Value=2^3  OutDataTypeStr=single
  B42 : Constant  Value=2^4  OutDataTypeStr=single
  B43 : Constant  Value=2^5  OutDataTypeStr=single
  B44 : Constant  Value=2^6  OutDataTypeStr=single
  B45 : Constant  Value=2^7  OutDataTypeStr=single
  B46 : Constant  Value=2^8  OutDataTypeStr=single
  B47 : Constant  Value=2^9  OutDataTypeStr=single
  B48 : Constant  Value=2^10  OutDataTypeStr=single
  B49 : Constant  Value=2^11  OutDataTypeStr=single
  B50 : Constant  OutDataTypeStr=single
  De-serialize : Subsystem
  NOT{,1..11} (12 alike) : Logic  Operator=NOT  IconShape=distinctive  AllPortsSameDT=off  OutDataTypeStr=boolean
  Product{32..43} (12 alike) : Product
  Out1 : Outport
  Out2 : Outport  Port=2
  Out3 : Outport  Port=3
  Out4 : Outport  Port=4
  Out5 : Outport  Port=5
  Out6 : Outport  Port=6
  Out7 : Outport  Port=7
  Out8 : Outport  Port=8
  Out9 : Outport  Port=9
  Out10 : Outport  Port=10
  Out11 : Outport  Port=11
  Out12 : Outport  Port=12
  wires:
  B42/1 -> Product36/1
  Add6/1 -> De-serialize/1(In1)
  B43/1 -> Product37/1
  NOT/1 -> Product32/2
  Product33/1 -> Add5/2
  Product36/1 -> Add5/5
  NOT11/1 -> Product43/2
  NOT6/1 -> Product38/2
  NOT1/1 -> Product33/2
  In5/1 -> NOT4/1
  Product37/1 -> Add5/6
  Product40/1 -> Add5/9
  B40/1 -> Product34/1
  De-serialize/2(Out2) -> Out2/1
  In9/1 -> NOT8/1
  NOT7/1 -> Product39/2
  B46/1 -> Product40/1
  Add5/1 -> Add6/1
  In1/1 -> NOT/1
  In12/1 -> NOT11/1
  Product43/1 -> Add5/12
  In6/1 -> NOT5/1
  B44/1 -> Product38/1
  In2/1 -> NOT1/1
  NOT2/1 -> Product34/2
  NOT4/1 -> Product36/2
  B41/1 -> Product35/1
  Product34/1 -> Add5/3
  De-serialize/10(Out10) -> Out10/1
  De-serialize/7(Out8) -> Out7/1
  Product42/1 -> Add5/11
  De-serialize/11(Out11) -> Out11/1
  In8/1 -> NOT7/1
  In11/1 -> NOT10/1
  In4/1 -> NOT3/1
  NOT10/1 -> Product42/2
  Product41/1 -> Add5/10
  De-serialize/12(Out12) -> Out12/1
  B48/1 -> Product42/1
  Product32/1 -> Add5/1
  B49/1 -> Product43/1
  Product38/1 -> Add5/7
  NOT9/1 -> Product41/2
  B38/1 -> Product32/1
  NOT8/1 -> Product40/2
  B50/1 -> Add6/2
  Product39/1 -> Add5/8
  NOT5/1 -> Product37/2
  NOT3/1 -> Product35/2
  De-serialize/8(Out5) -> Out8/1
  B47/1 -> Product41/1
  De-serialize/9(Out9) -> Out9/1
  Product35/1 -> Add5/4
  B39/1 -> Product33/1
  In10/1 -> NOT9/1
  B45/1 -> Product39/1
  In7/1 -> NOT6/1
  In3/1 -> NOT2/1
  De-serialize/4(Out4) -> Out4/1
  De-serialize/3(Out3) -> Out3/1
  De-serialize/5(Out6) -> Out5/1
  De-serialize/1(Out1) -> Out1/1
  De-serialize/6(Out7) -> Out6/1

== system ARINC429_BNR/Encoder/base 8 encoder ==
  In1 : Inport
  In2 : Inport  Port=2
  In3 : Inport  Port=3
  Subsystem : Subsystem
  Subsystem1 : Subsystem
  Subsystem2 : Subsystem
  Out1 : Outport
  Out2 : Outport  Port=2
  Out3 : Outport  Port=3
  Out4 : Outport  Port=4
  Out5 : Outport  Port=5
  Out6 : Outport  Port=6
  Out7 : Outport  Port=7
  Out8 : Outport  Port=8
  wires:
  In2/1 -> Subsystem1/1(In1)
  In1/1 -> Subsystem2/1(In1)
  In3/1 -> Subsystem/1(In1)
  Subsystem2/1(Out1) -> Out1/1
  Subsystem2/2(Out2) -> Out2/1
  Subsystem1/1(Out1) -> Out4/1
  Subsystem1/2(Out2) -> Out5/1
  Subsystem/1(Out1) -> Out7/1
  Subsystem/2(Out2) -> Out8/1
  Subsystem2/3(Out3) -> Out3/1
  Subsystem1/3(Out3) -> Out6/1

== system ARINC429_BNR/Decoder/De-serialize/Subsystem ==
  In1 : Inport
  Data Type Conversion5 : DataTypeConversion  OutDataTypeStr=uint32
  Data Type Conversion9 : DataTypeConversion  OutDataTypeStr=uint32
  Divide12 : Product  Inputs=*/  OutDataTypeStr=double
  Divide13 : Product  Inputs=*/  OutDataTypeStr=uint32
  Float Const : Constant  Value=2  OutDataTypeStr=single
  Float Const6 : Constant  Value=0.5  OutDataTypeStr=single
  Subtract5 : Sum  Inputs=+-
  Out1 : Outport
  Out2 : Outport  Port=2
  wires:
  Float Const/1 -> [F_2]
  Divide12/1 -> Subtract5/1, Data Type Conversion5/1
  Divide13/1 -> Data Type Conversion9/1
  Float Const6/1 -> Divide13/2
  Data Type Conversion5/1 -> Out2/1, Subtract5/2
  [F_2] -> Divide12/2
  Subtract5/1 -> Divide13/1
  Data Type Conversion9/1 -> Out1/1
  In1/1 -> Divide12/1

== system ARINC429_BNR/Decoder/De-serialize/Subsystem1 ==
  In1 : Inport
  Data Type Conversion5 : DataTypeConversion  OutDataTypeStr=uint32
  Data Type Conversion9 : DataTypeConversion  OutDataTypeStr=uint32
  Divide12 : Product  Inputs=*/  OutDataTypeStr=double
  Divide13 : Product  Inputs=*/  OutDataTypeStr=uint32
  Float Const : Constant  Value=2  OutDataTypeStr=single
  Float Const6 : Constant  Value=0.5  OutDataTypeStr=single
  Subtract5 : Sum  Inputs=+-
  Out1 : Outport
  Out2 : Outport  Port=2
  wires:
  Float Const/1 -> [F_2]
  Divide12/1 -> Subtract5/1, Data Type Conversion5/1
  Divide13/1 -> Data Type Conversion9/1
  Float Const6/1 -> Divide13/2
  Data Type Conversion5/1 -> Out2/1, Subtract5/2
  [F_2] -> Divide12/2
  Subtract5/1 -> Divide13/1
  Data Type Conversion9/1 -> Out1/1
  In1/1 -> Divide12/1

== system ARINC429_BNR/Decoder/De-serialize/Subsystem10 ==
  In1 : Inport
  Data Type Conversion5 : DataTypeConversion  OutDataTypeStr=uint32
  Data Type Conversion9 : DataTypeConversion  OutDataTypeStr=uint32
  Divide12 : Product  Inputs=*/  OutDataTypeStr=double
  Divide13 : Product  Inputs=*/  OutDataTypeStr=uint32
  Float Const : Constant  Value=2  OutDataTypeStr=single
  Float Const6 : Constant  Value=0.5  OutDataTypeStr=single
  Subtract5 : Sum  Inputs=+-
  Out1 : Outport
  Out2 : Outport  Port=2
  wires:
  Float Const/1 -> [F_2]
  Divide12/1 -> Subtract5/1, Data Type Conversion5/1
  Divide13/1 -> Data Type Conversion9/1
  Float Const6/1 -> Divide13/2
  Data Type Conversion5/1 -> Out2/1, Subtract5/2
  [F_2] -> Divide12/2
  Subtract5/1 -> Divide13/1
  Data Type Conversion9/1 -> Out1/1
  In1/1 -> Divide12/1

== system ARINC429_BNR/Decoder/De-serialize/Subsystem11 ==
  In1 : Inport
  Data Type Conversion5 : DataTypeConversion  OutDataTypeStr=uint32
  Data Type Conversion9 : DataTypeConversion  OutDataTypeStr=uint32
  Divide12 : Product  Inputs=*/  OutDataTypeStr=double
  Divide13 : Product  Inputs=*/  OutDataTypeStr=uint32
  Float Const : Constant  Value=2  OutDataTypeStr=single
  Float Const6 : Constant  Value=0.5  OutDataTypeStr=single
  Subtract5 : Sum  Inputs=+-
  Out1 : Outport
  Out2 : Outport  Port=2
  wires:
  Float Const/1 -> [F_2]
  Divide12/1 -> Subtract5/1, Data Type Conversion5/1
  Divide13/1 -> Data Type Conversion9/1
  Float Const6/1 -> Divide13/2
  Data Type Conversion5/1 -> Out2/1, Subtract5/2
  [F_2] -> Divide12/2
  Subtract5/1 -> Divide13/1
  Data Type Conversion9/1 -> Out1/1
  In1/1 -> Divide12/1

== system ARINC429_BNR/Decoder/De-serialize/Subsystem12 ==
  In1 : Inport
  Data Type Conversion5 : DataTypeConversion  OutDataTypeStr=uint32
  Data Type Conversion9 : DataTypeConversion  OutDataTypeStr=uint32
  Divide12 : Product  Inputs=*/  OutDataTypeStr=double
  Divide13 : Product  Inputs=*/  OutDataTypeStr=uint32
  Float Const : Constant  Value=2  OutDataTypeStr=single
  Float Const6 : Constant  Value=0.5  OutDataTypeStr=single
  Subtract5 : Sum  Inputs=+-
  Out1 : Outport
  Out2 : Outport  Port=2
  wires:
  Float Const/1 -> [F_2]
  Divide12/1 -> Subtract5/1, Data Type Conversion5/1
  Divide13/1 -> Data Type Conversion9/1
  Float Const6/1 -> Divide13/2
  Data Type Conversion5/1 -> Out2/1, Subtract5/2
  [F_2] -> Divide12/2
  Subtract5/1 -> Divide13/1
  Data Type Conversion9/1 -> Out1/1
  In1/1 -> Divide12/1

== system ARINC429_BNR/Decoder/De-serialize/Subsystem13 ==
  In1 : Inport
  Data Type Conversion5 : DataTypeConversion  OutDataTypeStr=uint32
  Data Type Conversion9 : DataTypeConversion  OutDataTypeStr=uint32
  Divide12 : Product  Inputs=*/  OutDataTypeStr=double
  Divide13 : Product  Inputs=*/  OutDataTypeStr=uint32
  Float Const : Constant  Value=2  OutDataTypeStr=single
  Float Const6 : Constant  Value=0.5  OutDataTypeStr=single
  Subtract5 : Sum  Inputs=+-
  Out1 : Outport
  Out2 : Outport  Port=2
  wires:
  Float Const/1 -> [F_2]
  Divide12/1 -> Subtract5/1, Data Type Conversion5/1
  Divide13/1 -> Data Type Conversion9/1
  Float Const6/1 -> Divide13/2
  Data Type Conversion5/1 -> Out2/1, Subtract5/2
  [F_2] -> Divide12/2
  Subtract5/1 -> Divide13/1
  Data Type Conversion9/1 -> Out1/1
  In1/1 -> Divide12/1

== system ARINC429_BNR/Decoder/De-serialize/Subsystem14 ==
  In1 : Inport
  Data Type Conversion5 : DataTypeConversion  OutDataTypeStr=uint32
  Data Type Conversion9 : DataTypeConversion  OutDataTypeStr=uint32
  Divide12 : Product  Inputs=*/  OutDataTypeStr=double
  Divide13 : Product  Inputs=*/  OutDataTypeStr=uint32
  Float Const : Constant  Value=2  OutDataTypeStr=single
  Float Const6 : Constant  Value=0.5  OutDataTypeStr=single
  Subtract5 : Sum  Inputs=+-
  Out1 : Outport
  Out2 : Outport  Port=2
  wires:
  Float Const/1 -> [F_2]
  Divide12/1 -> Subtract5/1, Data Type Conversion5/1
  Divide13/1 -> Data Type Conversion9/1
  Float Const6/1 -> Divide13/2
  Data Type Conversion5/1 -> Out2/1, Subtract5/2
  [F_2] -> Divide12/2
  Subtract5/1 -> Divide13/1
  Data Type Conversion9/1 -> Out1/1
  In1/1 -> Divide12/1

== system ARINC429_BNR/Decoder/De-serialize/Subsystem15 ==
  In1 : Inport
  Data Type Conversion5 : DataTypeConversion  OutDataTypeStr=uint32
  Data Type Conversion9 : DataTypeConversion  OutDataTypeStr=uint32
  Divide12 : Product  Inputs=*/  OutDataTypeStr=double
  Divide13 : Product  Inputs=*/  OutDataTypeStr=uint32
  Float Const : Constant  Value=2  OutDataTypeStr=single
  Float Const6 : Constant  Value=0.5  OutDataTypeStr=single
  Subtract5 : Sum  Inputs=+-
  Out1 : Outport
  Out2 : Outport  Port=2
  wires:
  Float Const/1 -> [F_2]
  Divide12/1 -> Subtract5/1, Data Type Conversion5/1
  Divide13/1 -> Data Type Conversion9/1
  Float Const6/1 -> Divide13/2
  Data Type Conversion5/1 -> Out2/1, Subtract5/2
  [F_2] -> Divide12/2
  Subtract5/1 -> Divide13/1
  Data Type Conversion9/1 -> Out1/1
  In1/1 -> Divide12/1

== system ARINC429_BNR/Decoder/De-serialize/Subsystem16 ==
  In1 : Inport
  Data Type Conversion5 : DataTypeConversion  OutDataTypeStr=uint32
  Data Type Conversion9 : DataTypeConversion  OutDataTypeStr=uint32
  Divide12 : Product  Inputs=*/  OutDataTypeStr=double
  Divide13 : Product  Inputs=*/  OutDataTypeStr=uint32
  Float Const : Constant  Value=2  OutDataTypeStr=single
  Float Const6 : Constant  Value=0.5  OutDataTypeStr=single
  Subtract5 : Sum  Inputs=+-
  Out1 : Outport
  Out2 : Outport  Port=2
  wires:
  Float Const/1 -> [F_2]
  Divide12/1 -> Subtract5/1, Data Type Conversion5/1
  Divide13/1 -> Data Type Conversion9/1
  Float Const6/1 -> Divide13/2
  Data Type Conversion5/1 -> Out2/1, Subtract5/2
  [F_2] -> Divide12/2
  Subtract5/1 -> Divide13/1
  Data Type Conversion9/1 -> Out1/1
  In1/1 -> Divide12/1

== system ARINC429_BNR/Decoder/De-serialize/Subsystem17 ==
  In1 : Inport
  Data Type Conversion5 : DataTypeConversion  OutDataTypeStr=uint32
  Data Type Conversion9 : DataTypeConversion  OutDataTypeStr=uint32
  Divide12 : Product  Inputs=*/  OutDataTypeStr=double
  Divide13 : Product  Inputs=*/  OutDataTypeStr=uint32
  Float Const : Constant  Value=2  OutDataTypeStr=single
  Float Const6 : Constant  Value=0.5  OutDataTypeStr=single
  Subtract5 : Sum  Inputs=+-
  Out1 : Outport
  Out2 : Outport  Port=2
  wires:
  Float Const/1 -> [F_2]
  Divide12/1 -> Subtract5/1, Data Type Conversion5/1
  Divide13/1 -> Data Type Conversion9/1
  Float Const6/1 -> Divide13/2
  Data Type Conversion5/1 -> Out2/1, Subtract5/2
  [F_2] -> Divide12/2
  Subtract5/1 -> Divide13/1
  Data Type Conversion9/1 -> Out1/1
  In1/1 -> Divide12/1

== system ARINC429_BNR/Decoder/De-serialize/Subsystem18 ==
  In1 : Inport
  Data Type Conversion5 : DataTypeConversion  OutDataTypeStr=uint32
  Data Type Conversion9 : DataTypeConversion  OutDataTypeStr=uint32
  Divide12 : Product  Inputs=*/
  Divide13 : Product  Inputs=*/  OutDataTypeStr=uint32
  Float Const : Constant  Value=2  OutDataTypeStr=single
  Float Const6 : Constant  Value=0.5  OutDataTypeStr=single
  Subtract5 : Sum  Inputs=+-
  Out1 : Outport
  Out2 : Outport  Port=2
  wires:
  Float Const/1 -> [F_2]
  Divide12/1 -> Subtract5/1, Data Type Conversion5/1
  Divide13/1 -> Data Type Conversion9/1
  Float Const6/1 -> Divide13/2
  Data Type Conversion5/1 -> Out2/1, Subtract5/2
  [F_2] -> Divide12/2
  Subtract5/1 -> Divide13/1
  Data Type Conversion9/1 -> Out1/1
  In1/1 -> Divide12/1

== system ARINC429_BNR/Decoder/De-serialize/Subsystem19 ==
  In1 : Inport
  Data Type Conversion5 : DataTypeConversion  OutDataTypeStr=uint32
  Data Type Conversion9 : DataTypeConversion  OutDataTypeStr=uint32
  Divide12 : Product  Inputs=*/
  Divide13 : Product  Inputs=*/  OutDataTypeStr=uint32
  Float Const : Constant  Value=2  OutDataTypeStr=single
  Float Const6 : Constant  Value=0.5  OutDataTypeStr=single
  Subtract5 : Sum  Inputs=+-
  Out1 : Outport
  Out2 : Outport  Port=2
  wires:
  Float Const/1 -> [F_2]
  Divide12/1 -> Subtract5/1, Data Type Conversion5/1
  Divide13/1 -> Data Type Conversion9/1
  Float Const6/1 -> Divide13/2
  Data Type Conversion5/1 -> Out2/1, Subtract5/2
  [F_2] -> Divide12/2
  Subtract5/1 -> Divide13/1
  Data Type Conversion9/1 -> Out1/1
  In1/1 -> Divide12/1

== system ARINC429_BNR/Decoder/De-serialize/Subsystem2 ==
  In1 : Inport
  Data Type Conversion5 : DataTypeConversion  OutDataTypeStr=uint32
  Data Type Conversion9 : DataTypeConversion  OutDataTypeStr=uint32
  Divide12 : Product  Inputs=*/  OutDataTypeStr=double
  Divide13 : Product  Inputs=*/  OutDataTypeStr=uint32
  Float Const : Constant  Value=2  OutDataTypeStr=single
  Float Const6 : Constant  Value=0.5  OutDataTypeStr=single
  Subtract5 : Sum  Inputs=+-
  Out1 : Outport
  Out2 : Outport  Port=2
  wires:
  Float Const/1 -> [F_2]
  Divide12/1 -> Subtract5/1, Data Type Conversion5/1
  Divide13/1 -> Data Type Conversion9/1
  Float Const6/1 -> Divide13/2
  Data Type Conversion5/1 -> Out2/1, Subtract5/2
  [F_2] -> Divide12/2
  Subtract5/1 -> Divide13/1
  Data Type Conversion9/1 -> Out1/1
  In1/1 -> Divide12/1

== system ARINC429_BNR/Decoder/De-serialize/Subsystem20 ==
  In1 : Inport
  Data Type Conversion5 : DataTypeConversion  OutDataTypeStr=uint32
  Data Type Conversion9 : DataTypeConversion  OutDataTypeStr=uint32
  Divide12 : Product  Inputs=*/
  Divide13 : Product  Inputs=*/  OutDataTypeStr=uint32
  Float Const : Constant  Value=2  OutDataTypeStr=single
  Float Const6 : Constant  Value=0.5  OutDataTypeStr=single
  Subtract5 : Sum  Inputs=+-
  Out1 : Outport
  Out2 : Outport  Port=2
  wires:
  Float Const/1 -> [F_2]
  Divide12/1 -> Subtract5/1, Data Type Conversion5/1
  Divide13/1 -> Data Type Conversion9/1
  Float Const6/1 -> Divide13/2
  Data Type Conversion5/1 -> Out2/1, Subtract5/2
  [F_2] -> Divide12/2
  Subtract5/1 -> Divide13/1
  Data Type Conversion9/1 -> Out1/1
  In1/1 -> Divide12/1

== system ARINC429_BNR/Decoder/De-serialize/Subsystem21 ==
  In1 : Inport
  Data Type Conversion5 : DataTypeConversion  OutDataTypeStr=uint32
  Data Type Conversion9 : DataTypeConversion  OutDataTypeStr=uint32
  Divide12 : Product  Inputs=*/
  Divide13 : Product  Inputs=*/  OutDataTypeStr=uint32
  Float Const : Constant  Value=2  OutDataTypeStr=single
  Float Const6 : Constant  Value=0.5  OutDataTypeStr=single
  Subtract5 : Sum  Inputs=+-
  Out1 : Outport
  Out2 : Outport  Port=2
  wires:
  Float Const/1 -> [F_2]
  Divide12/1 -> Subtract5/1, Data Type Conversion5/1
  Divide13/1 -> Data Type Conversion9/1
  Float Const6/1 -> Divide13/2
  Data Type Conversion5/1 -> Out2/1, Subtract5/2
  [F_2] -> Divide12/2
  Subtract5/1 -> Divide13/1
  Data Type Conversion9/1 -> Out1/1
  In1/1 -> Divide12/1

== system ARINC429_BNR/Decoder/De-serialize/Subsystem22 ==
  In1 : Inport
  Data Type Conversion5 : DataTypeConversion  OutDataTypeStr=uint32
  Data Type Conversion9 : DataTypeConversion  OutDataTypeStr=uint32
  Divide12 : Product  Inputs=*/
  Divide13 : Product  Inputs=*/  OutDataTypeStr=uint32
  Float Const : Constant  Value=2  OutDataTypeStr=single
  Float Const6 : Constant  Value=0.5  OutDataTypeStr=single
  Subtract5 : Sum  Inputs=+-
  Out1 : Outport
  Out2 : Outport  Port=2
  wires:
  Float Const/1 -> [F_2]
  Divide12/1 -> Subtract5/1, Data Type Conversion5/1
  Divide13/1 -> Data Type Conversion9/1
  Float Const6/1 -> Divide13/2
  Data Type Conversion5/1 -> Out2/1, Subtract5/2
  [F_2] -> Divide12/2
  Subtract5/1 -> Divide13/1
  Data Type Conversion9/1 -> Out1/1
  In1/1 -> Divide12/1

== system ARINC429_BNR/Decoder/De-serialize/Subsystem23 ==
  In1 : Inport
  Data Type Conversion5 : DataTypeConversion  OutDataTypeStr=uint32
  Data Type Conversion9 : DataTypeConversion  OutDataTypeStr=uint32
  Divide12 : Product  Inputs=*/
  Divide13 : Product  Inputs=*/  OutDataTypeStr=uint32
  Float Const : Constant  Value=2  OutDataTypeStr=single
  Float Const6 : Constant  Value=0.5  OutDataTypeStr=single
  Subtract5 : Sum  Inputs=+-
  Out1 : Outport
  Out2 : Outport  Port=2
  wires:
  Float Const/1 -> [F_2]
  Divide12/1 -> Subtract5/1, Data Type Conversion5/1
  Divide13/1 -> Data Type Conversion9/1
  Float Const6/1 -> Divide13/2
  Data Type Conversion5/1 -> Out2/1, Subtract5/2
  [F_2] -> Divide12/2
  Subtract5/1 -> Divide13/1
  Data Type Conversion9/1 -> Out1/1
  In1/1 -> Divide12/1

== system ARINC429_BNR/Decoder/De-serialize/Subsystem24 ==
  In1 : Inport
  Data Type Conversion5 : DataTypeConversion  OutDataTypeStr=uint32
  Data Type Conversion9 : DataTypeConversion  OutDataTypeStr=uint32
  Divide12 : Product  Inputs=*/
  Divide13 : Product  Inputs=*/  OutDataTypeStr=uint32
  Float Const : Constant  Value=2  OutDataTypeStr=single
  Float Const6 : Constant  Value=0.5  OutDataTypeStr=single
  Subtract5 : Sum  Inputs=+-
  Out1 : Outport
  Out2 : Outport  Port=2
  wires:
  Float Const/1 -> [F_2]
  Divide12/1 -> Subtract5/1, Data Type Conversion5/1
  Divide13/1 -> Data Type Conversion9/1
  Float Const6/1 -> Divide13/2
  Data Type Conversion5/1 -> Out2/1, Subtract5/2
  [F_2] -> Divide12/2
  Subtract5/1 -> Divide13/1
  Data Type Conversion9/1 -> Out1/1
  In1/1 -> Divide12/1

== system ARINC429_BNR/Decoder/De-serialize/Subsystem25 ==
  In1 : Inport
  Data Type Conversion5 : DataTypeConversion  OutDataTypeStr=uint32
  Data Type Conversion9 : DataTypeConversion  OutDataTypeStr=uint32
  Divide12 : Product  Inputs=*/
  Divide13 : Product  Inputs=*/  OutDataTypeStr=uint32
  Float Const : Constant  Value=2  OutDataTypeStr=single
  Float Const6 : Constant  Value=0.5  OutDataTypeStr=single
  Subtract5 : Sum  Inputs=+-
  Out1 : Outport
  Out2 : Outport  Port=2
  wires:
  Float Const/1 -> [F_2]
  Divide12/1 -> Subtract5/1, Data Type Conversion5/1
  Divide13/1 -> Data Type Conversion9/1
  Float Const6/1 -> Divide13/2
  Data Type Conversion5/1 -> Out2/1, Subtract5/2
  [F_2] -> Divide12/2
  Subtract5/1 -> Divide13/1
  Data Type Conversion9/1 -> Out1/1
  In1/1 -> Divide12/1

== system ARINC429_BNR/Decoder/De-serialize/Subsystem26 ==
  In1 : Inport
  Data Type Conversion5 : DataTypeConversion  OutDataTypeStr=uint32
  Data Type Conversion9 : DataTypeConversion  OutDataTypeStr=uint32
  Divide12 : Product  Inputs=*/
  Divide13 : Product  Inputs=*/  OutDataTypeStr=uint32
  Float Const : Constant  Value=2  OutDataTypeStr=single
  Float Const6 : Constant  Value=0.5  OutDataTypeStr=single
  Subtract5 : Sum  Inputs=+-
  Out1 : Outport
  Out2 : Outport  Port=2
  wires:
  Float Const/1 -> [F_2]
  Divide12/1 -> Subtract5/1, Data Type Conversion5/1
  Divide13/1 -> Data Type Conversion9/1
  Float Const6/1 -> Divide13/2
  Data Type Conversion5/1 -> Out2/1, Subtract5/2
  [F_2] -> Divide12/2
  Subtract5/1 -> Divide13/1
  Data Type Conversion9/1 -> Out1/1
  In1/1 -> Divide12/1

== system ARINC429_BNR/Decoder/De-serialize/Subsystem27 ==
  In1 : Inport
  Data Type Conversion5 : DataTypeConversion  OutDataTypeStr=uint32
  Data Type Conversion9 : DataTypeConversion  OutDataTypeStr=uint32
  Divide12 : Product  Inputs=*/
  Divide13 : Product  Inputs=*/  OutDataTypeStr=uint32
  Float Const : Constant  Value=2  OutDataTypeStr=single
  Float Const6 : Constant  Value=0.5  OutDataTypeStr=single
  Subtract5 : Sum  Inputs=+-
  Out1 : Outport
  Out2 : Outport  Port=2
  wires:
  Float Const/1 -> [F_2]
  Divide12/1 -> Subtract5/1, Data Type Conversion5/1
  Divide13/1 -> Data Type Conversion9/1
  Float Const6/1 -> Divide13/2
  Data Type Conversion5/1 -> Out2/1, Subtract5/2
  [F_2] -> Divide12/2
  Subtract5/1 -> Divide13/1
  Data Type Conversion9/1 -> Out1/1
  In1/1 -> Divide12/1

== system ARINC429_BNR/Decoder/De-serialize/Subsystem28 ==
  In1 : Inport
  Data Type Conversion5 : DataTypeConversion  OutDataTypeStr=uint32
  Data Type Conversion9 : DataTypeConversion  OutDataTypeStr=uint32
  Divide12 : Product  Inputs=*/
  Divide13 : Product  Inputs=*/  OutDataTypeStr=uint32
  Float Const : Constant  Value=2  OutDataTypeStr=single
  Float Const6 : Constant  Value=0.5  OutDataTypeStr=single
  Subtract5 : Sum  Inputs=+-
  Out1 : Outport
  Out2 : Outport  Port=2
  wires:
  Float Const/1 -> [F_2]
  Divide12/1 -> Subtract5/1, Data Type Conversion5/1
  Divide13/1 -> Data Type Conversion9/1
  Float Const6/1 -> Divide13/2
  Data Type Conversion5/1 -> Out2/1, Subtract5/2
  [F_2] -> Divide12/2
  Subtract5/1 -> Divide13/1
  Data Type Conversion9/1 -> Out1/1
  In1/1 -> Divide12/1
